simulink model "dcm"  (R2020b)
settings: Solver=VariableStepAuto  StartTime=0.0  StopTime=10.0  RelTol=1e-3
settings Model: Creator=whitehole  LastModifiedBy=whitehole

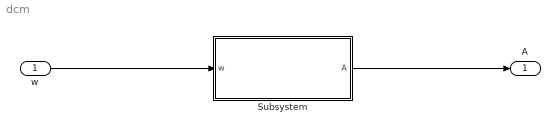
== system dcm ==
  w : Inport
  Subsystem : Subsystem
  A : Outport
  wires:
  w/1 -> Subsystem/1(w)
  Subsystem/1(A) -> A/1

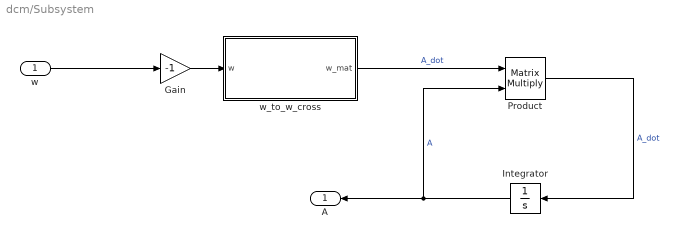
== system dcm/Subsystem ==
  w : Inport
  Gain : Gain  Gain=-1
  Integrator : Integrator  InitialCondition=eye(3)
  Product : Product  Multiplication=Matrix(*)
  w_to_w_cross : Subsystem
  A : Outport
  wires:
  w/1 -> Gain/1
  Gain/1 -> w_to_w_cross/1(w)
  Product/1 -> Integrator/1  "A_dot"
  w_to_w_cross/1(w_mat) -> Product/1  "A_dot"
  Integrator/1 -> A/1, Product/2  "A"

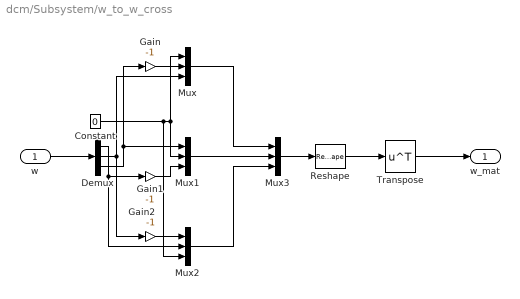
== system dcm/Subsystem/w_to_w_cross ==
  w : Inport
  Constant : Constant  Value=0
  Demux : Demux  Outputs=3
  Gain : Gain  Gain=-1
  Gain1 : Gain  Gain=-1
  Gain2 : Gain  Gain=-1
  Mux{,1..3} (4 alike) : Mux  Inputs=3
  Reshape : Reshape  OutputDimensionality=Customize  OutputDimensions=[3,3]
  Transpose : Math  Operator=transpose  SaturateOnIntegerOverflow=on
  w_mat : Outport
  wires:
  Reshape/1 -> Transpose/1
  Gain/1 -> Mux/2
  Gain1/1 -> Mux1/3
  Mux1/1 -> Mux3/2
  Mux/1 -> Mux3/1
  Demux/1 -> Mux2/2, Gain1/1
  Transpose/1 -> w_mat/1
  Gain2/1 -> Mux2/1
  Mux2/1 -> Mux3/3
  Mux3/1 -> Reshape/1
  Constant/1 -> Mux/1, Mux1/2, Mux2/3
  w/1 -> Demux/1
  Demux/2 -> Mux/3, Gain2/1
  Demux/3 -> Mux1/1, Gain/1
